simulink model "quatro_b"  (R2015a)
settings: Solver=ode45  StartTime=0.0  StopTime=10.0  RelTol=1e-3
undefined symbols (not defined in the file or in its folder): K
settings Model: Creator=joao  LastModifiedBy=João F
settings DataIOCC: SignalLoggingSaveFormat=ModelDataLogs
settings OptimizationCC: ExpressionDepthLimit=2147483647
settings DebuggingCC: UnderspecifiedInitializationDetection=Classic  MergeDetectMultiDrivingBlocksExec=none  SolverPrmCheckMsg=warning  FcnCallInpInsideContextMsg=EnableAllAsWarning  StateNameClashWarn=warning
settings GRTTargetCC: CombineOutputUpdateFcns=off  GRTInterface=on

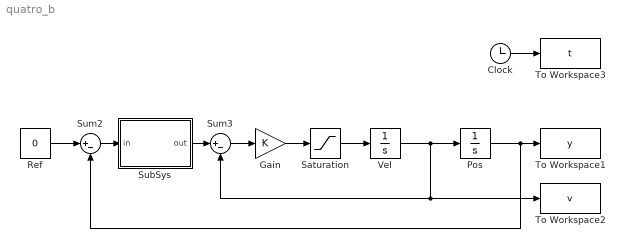
== system quatro_b ==
  Clock : Clock
  Gain : Gain  Gain=K
  Pos : Integrator  InitialCondition=1
  Ref : Constant  Value=0
  Saturation : Saturate
  SubSys : MATLAB Function  TreatAsAtomicUnit=on
  Sum2 : Sum  Inputs=|+-
  Sum3 : Sum  Inputs=|+-
  To Workspace1 : ToWorkspace  VariableName=y  SampleTime=-1
  To Workspace2 : ToWorkspace  VariableName=v  SampleTime=-1
  To Workspace3 : ToWorkspace  VariableName=t  SampleTime=-1
  Vel : Integrator
  wires:
  Pos/1 -> Sum2/2, To Workspace1/1
  Vel/1 -> Pos/1, Sum3/2, To Workspace2/1
  Saturation/1 -> Vel/1
  Gain/1 -> Saturation/1
  Sum3/1 -> Gain/1
  Clock/1 -> To Workspace3/1
  Ref/1 -> Sum2/1
  Sum2/1 -> SubSys/1(in)
  SubSys/1(out) -> Sum3/1

== matlab function quatro_b/SubSys ==
  data: in input; out output
function out = f(in)

out = sign(in)*sqrt(2*abs(in));
